simulink model "WPT_LCC_S_48V_2016b"  (R2023b)
settings: Solver=FixedStepAuto  StartTime=0.0  StopTime=0.02  FixedStep=0.1e-6  MaxStep=1e-6  RelTol=1e-3
libraries: spsSeriesRLCBranchLib x8, spsCurrentMeasurementLib x4, spsDiodeLib x4, spsMosfetLib x4, spsMultimeterLib x4, spsVoltageMeasurementLib x4, simulink x2, spsIdealSwitchLib x2, spsMutualInductanceLib x1, spsRMSLib x1, spsDCVoltageSourceLib x1, sps_lib x1
settings Model: Creator=Admin  LastModifiedBy=smith
settings SolverCC: AlgebraicLoopSolver=TrustRegion
settings DebuggingCC: ArithmeticOperatorsInVariantConditions=warning
settings SFSimCC: CustomCodeUndefinedFunction=UseInterfaceOnly
settings CodeAppCC: StateflowObjectComments=on

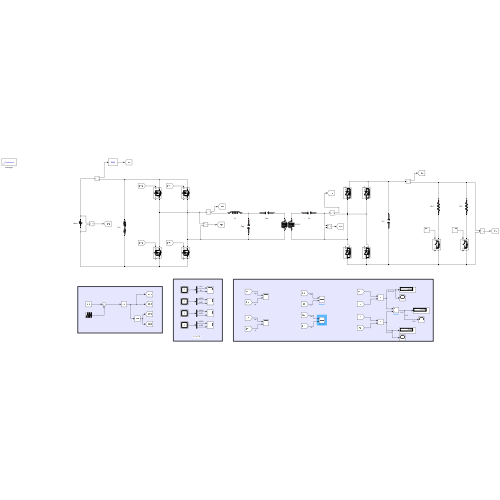
[thumbnail: Simulink's stored preview of the top-level diagram]
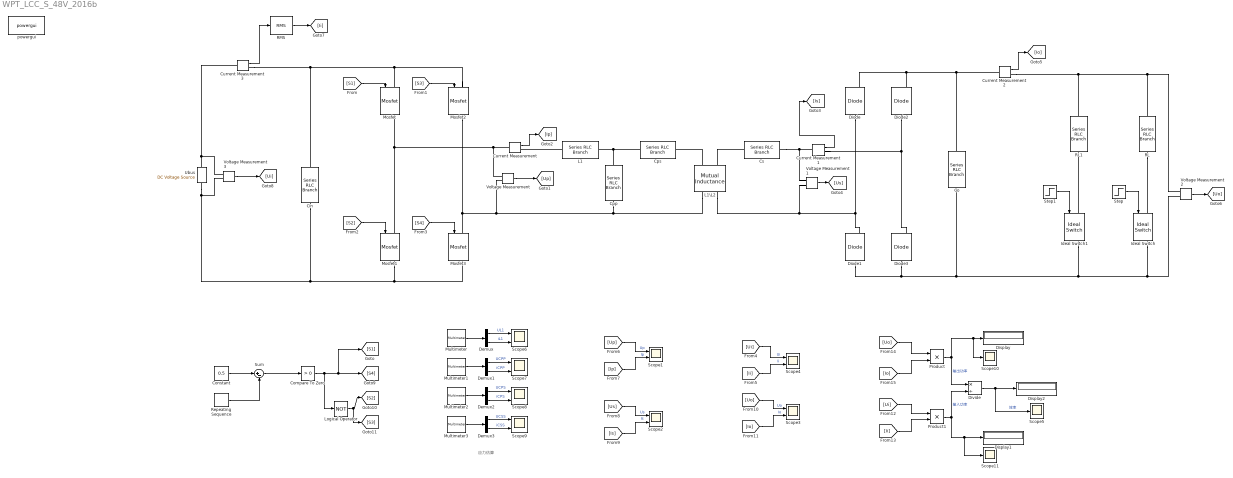
== system WPT_LCC_S_48V_2016b ==
  note: 应力估算
  Cin : spsSeriesRLCBranchLib/Series RLC Branch  LConnTagsString=__new0  RConnTagsString=__new0  BranchType=RC  Resistance=0.020  Inductance=1e-3  SetiL0=off  InitialCurrent=0  Capacitance=100e-6  Setx0=on  InitialVoltage=48  Measurements=None
  Co : spsSeriesRLCBranchLib/Series RLC Branch  LConnTagsString=__new0  RConnTagsString=__new0  BranchType=C  Resistance=1  Inductance=1e-3  SetiL0=off  InitialCurrent=0  Capacitance=100e-6  Setx0=off  InitialVoltage=0  Measurements=None
  Compare To Zero : simulink/Logic and Bit Operations/Compare To Zero  relop=>  OutDataTypeStr=boolean
  Constant : Constant  Value=0.5
  Cpp : spsSeriesRLCBranchLib/Series RLC Branch  LConnTagsString=__new0  RConnTagsString=__new0  BranchType=C  Resistance=1  Inductance=1e-3  SetiL0=off  InitialCurrent=0  Capacitance=202.96213e-9  Setx0=off  InitialVoltage=0  Measurements=Branch voltage and current
  Cps : spsSeriesRLCBranchLib/Series RLC Branch  LConnTagsString=__new0  RConnTagsString=__new0  BranchType=C  Resistance=1  Inductance=1e-3  SetiL0=off  InitialCurrent=0  Capacitance=144.58184e-9  Setx0=off  InitialVoltage=0  Measurements=Branch voltage and current
  Cs : spsSeriesRLCBranchLib/Series RLC Branch  LConnTagsString=__new0  RConnTagsString=__new0  BranchType=C  Resistance=1  Inductance=1e-3  SetiL0=off  InitialCurrent=0  Capacitance=100.43432e-9  Setx0=off  InitialVoltage=0  Measurements=Branch voltage and current
  Current Measurement{,1..3} (4 alike) : spsCurrentMeasurementLib/Current Measurement  PhasorSimulation=off  OutputType=Complex  PSBequivalent=0
  Demux{,1..3} (4 alike) : Demux  Outputs=2
  Diode{,1..3} (4 alike) : spsDiodeLib/Diode  Ron=0.001  Lon=0  Vf=0.8  IC=0  UseSnubber=0  Rs=500  Cs=250e-9  Measurements=on
  Display : Display
  Display1 : Display
  Display2 : Display
  Divide : Product  Inputs=*/
  Ideal Switch : spsIdealSwitchLib/Ideal Switch  Ron=0.001  Lon=0  IC=0  Rs=1e5  Cs=inf  Measurements=on
  Ideal Switch1 : spsIdealSwitchLib/Ideal Switch  Ron=0.001  Lon=0  IC=0  Rs=1e5  Cs=inf  Measurements=on
  L1 : spsSeriesRLCBranchLib/Series RLC Branch  LConnTagsString=__new0  RConnTagsString=__new0  BranchType=L  Resistance=1  Inductance=12.480306e-6  SetiL0=off  InitialCurrent=0  Capacitance=116.864e-9  Setx0=off  InitialVoltage=0  Measurements=Branch voltage and current
  L1\L2 : spsMutualInductanceLib/Mutual Inductance  LConnTagsString=a|b  RConnTagsString=A|B  TypeOfMutual=Two or three windings with equal mutual terms  NumberOfWindings=3  SelfImpedance1=[0.1 30e-06]  SelfImpedance2=[0.1 30e-06]  ThreeWindings=off  SelfImpedance3=[ 1.1 1.1e-03]  MutualImpedance=[0.2 14e-06]  InductanceMatrix="[1.0 0.9  0.9 ;  0.9 1.0  0.9;  0.9 0.9 1.0 ] * 1e-3"  ResistanceMatrix="[1.0 0.9  0.9 ;  0.9 1.0  0.9;  0.9 0.9 1.0 ]"  Measurements=None
      settings: LibrarySourceBlock=sps_lib/Passives/Mutual Inductance
  Logical Operator : Logic  Operator=NOT  AllPortsSameDT=off  OutDataTypeStr=boolean
  Mosfet{,1..3} (4 alike) : spsMosfetLib/Mosfet  Ron=0.1  Lon=0  Rd=0.01  Vfd=0  IC=0  Rs=1e5  Cs=inf  Measurements=on
  Multimeter : spsMultimeterLib/Multimeter  L=8  sel=[4 8]  yselected={}  Gain=[1 1]  OutputType=Complex  PlotAtSimulationStop=off  PhasorSimulation=off
  Multimeter1 : spsMultimeterLib/Multimeter  L=8  sel=[1 5]  yselected={}  Gain=[1 1]  OutputType=Complex  PlotAtSimulationStop=off  PhasorSimulation=off
  Multimeter2 : spsMultimeterLib/Multimeter  L=8  sel=[2 6]  yselected={}  Gain=[1 1]  OutputType=Complex  PlotAtSimulationStop=off  PhasorSimulation=off
  Multimeter3 : spsMultimeterLib/Multimeter  L=8  sel=[3 7]  yselected={}  Gain=[1 1]  OutputType=Complex  PlotAtSimulationStop=off  PhasorSimulation=off
  Product : Product
  Product1 : Product
  RL : spsSeriesRLCBranchLib/Series RLC Branch  LConnTagsString=__new0  RConnTagsString=__new0  BranchType=R  Resistance=100  Inductance=1e-3  SetiL0=off  InitialCurrent=0  Capacitance=100e-6  Setx0=off  InitialVoltage=0  Measurements=None
  RL1 : spsSeriesRLCBranchLib/Series RLC Branch  LConnTagsString=__new0  RConnTagsString=__new0  BranchType=R  Resistance=99999999  Inductance=1e-3  SetiL0=off  InitialCurrent=0  Capacitance=100e-6  Setx0=off  InitialVoltage=0  Measurements=None
  RMS : spsRMSLib/RMS  TrueRMS=on  Freq=84000  RMSInit=0  Ts=0
  Repeating Sequence : simulink/Sources/Repeating Sequence  rep_seq_t=[0 1/84e3]  rep_seq_y=[0 1]
  Scope{1..4,6..9} (8 alike) : Scope  NumInputPorts=2
  Scope10 : Scope
  Scope11 : Scope
  Scope5 : Scope
  Step : Step  Time=0.01  SampleTime=0
  Step1 : Step  Time=0.01  Before=1  After=0  SampleTime=0
  Sum : Sum  Inputs=|+-
  Ubus : spsDCVoltageSourceLib/DC Voltage Source  Amplitude=24  Measurements=None
  Voltage Measurement{,1..3} (4 alike) : spsVoltageMeasurementLib/Voltage Measurement  PhasorSimulation=off  OutputType=Complex  PSBequivalent=0
  powergui : sps_lib/powergui  Priority=1  SimulationMode=Continuous  SampleTime=0.1e-6  frequency=60  Iterations=50  frequencyindice=0  Pbase=100e6  ErrMax=1e-4  UnitsV=kV  UnitsW=MW  buscounter=0  FunctionMessages=off  echomessages=off  EnableUseOfTLC=off  CurrentSourceSwitches=off  DisableSnubberDevices=off  DisableRonSwitches=off  DisableVfSwitches=off  DisplayEquations=off  AutomaticDiscreteSolvers=off  SolverType=Tustin/Backward Euler (TBE)  Interpol=off  ExternalGateDelay=off  methode=off  Ts=100  x0status=blocks  SPID=on  SwTol=0  HookPort=off  NonlinearTolerance=1e-4  nMaxIteration=100  ContinueOnMaxIteration=off  RestoreLinks=warning  ResistiveCurrentMeasurement=off  Frange=[0:2:500]  Ylog=off  Xlog=on  ShowGrid=off  save=off  variable=ZData  structure=0  ZoomFFT=off  StartTime=0.0  cycles=1  DisplayStyle=1  fundamental=60  FreqAxis=off  MaxFrequency=1000  frequencyindicesteady=1  RmsSteady=1  display=off
  wires:
  [S3] -> Mosfet2/1
  [S1] -> Mosfet/1
  [S2] -> Mosfet1/1
  [S4] -> Mosfet3/1
  Voltage Measurement/1 -> [Up]
  Current Measurement/1 -> [Ip]
  Voltage Measurement1/1 -> [Us]
  Current Measurement1/1 -> [Is]
  Voltage Measurement2/1 -> [Uo]
  Current Measurement2/1 -> [Io]
  Constant/1 -> Sum/1
  Repeating Sequence/1 -> Sum/2
  Sum/1 -> Compare To Zero/1
  Compare To Zero/1 -> [S4], [S1], Logical Operator/1
  Logical Operator/1 -> [S3], [S2]
  [Ip] -> Scope1/2  "Ip"
  [Up] -> Scope1/1  "Up"
  [Us] -> Scope2/1  "Us"
  [Is] -> Scope2/2  "Is"
  [Io] -> Scope3/2  "Io"
  [Uo] -> Scope3/1  "Uo"
  Product/1 -> Divide/1, Scope10/1, Display/1  "输出功率"
  Current Measurement3/1 -> RMS/1
  Voltage Measurement3/1 -> [Ui]
  RMS/1 -> [Ii]
  [Ui] -> Scope4/1  "Ui"
  [Ii] -> Scope4/2  "Ii"
  Product1/1 -> Divide/2, Scope11/1, Display1/1  "输入功率"
  [Uo] -> Product/1
  [Io] -> Product/2
  [Ii] -> Product1/2
  [Ui] -> Product1/1
  Divide/1 -> Scope5/1, Display2/1  "效率"
  Multimeter/1 -> Demux/1
  Demux/1 -> Scope6/1  "UL1"
  Demux/2 -> Scope6/2  "iL1"
  Demux1/2 -> Scope7/2  "iCPP"
  Demux1/1 -> Scope7/1  "UCPP"
  Multimeter1/1 -> Demux1/1
  Multimeter2/1 -> Demux2/1
  Demux2/1 -> Scope8/1  "UCPS"
  Demux2/2 -> Scope8/2  "iCPS"
  Demux3/2 -> Scope9/2  "iCSS"
  Demux3/1 -> Scope9/1  "UCSS"
  Multimeter3/1 -> Demux3/1
  Step/1 -> Ideal Switch/1
  Step1/1 -> Ideal Switch1/1
  connections:
  Mosfet1/LConn1 -- Voltage Measurement/LConn1 -- Current Measurement/LConn1 -- Mosfet/RConn1
  Mosfet2/RConn1 -- L1\L2/RConn1 -- Cpp/RConn1 -- Voltage Measurement/LConn2 -- Mosfet3/LConn1
  Mosfet1/RConn1 -- Voltage Measurement3/LConn2 -- Ubus/LConn1 -- Cin/RConn1 -- Mosfet3/RConn1
  L1\L2/LConn1 -- Cps/RConn1
  Diode/LConn1 -- Diode1/RConn1 -- Voltage Measurement1/LConn2 -- L1\L2/RConn2
  Diode2/LConn1 -- Diode3/RConn1 -- Current Measurement1/RConn1
  Cs/LConn1 -- L1\L2/LConn2
  Co/LConn1 -- Current Measurement2/LConn1 -- Diode2/RConn1 -- Diode/RConn1
  Diode3/LConn1 -- Diode1/LConn1 -- Ideal Switch1/RConn1 -- Ideal Switch/RConn1 -- Voltage Measurement2/LConn2 -- Co/RConn1
  Cs/RConn1 -- Voltage Measurement1/LConn1 -- Current Measurement1/LConn1
  Current Measurement2/RConn1 -- RL1/LConn1 -- RL/LConn1 -- Voltage Measurement2/LConn1
  Mosfet2/LConn1 -- Current Measurement3/RConn1 -- Cin/LConn1 -- Mosfet/LConn1
  Cps/LConn1 -- Cpp/LConn1 -- L1/RConn1
  L1/LConn1 -- Current Measurement/RConn1
  Voltage Measurement3/LConn1 -- Current Measurement3/LConn1 -- Ubus/RConn1
  RL/RConn1 -- Ideal Switch/LConn1
  Ideal Switch1/LConn1 -- RL1/RConn1
